simulink model "smib_attack_v2"  (Simulink 8.9)
settings: Solver=ode45  StartTime=0.0  StopTime=10  RelTol=1e-3  EnableMultiTasking=on
values from neighbouring files (symbols this model uses):
  delta0 = 1.1198    [smib_execution.m]
  omega0 = 0    [smib_execution.m]
libraries: simulink x1
settings Model: Creator=Luan Nguyen  LastModifiedBy=LuanNguyen
settings OptimizationCC: ExpressionDepthLimit=2147483647
settings DebuggingCC: MultiTaskDSMMsg=warning  MultiTaskCondExecSysMsg=none  FcnCallInpInsideContextMsg=error
settings GRTTargetCC: CombineOutputUpdateFcns=on  GRTInterface=off
settings ConfigComp: CovSFcnEnable=off

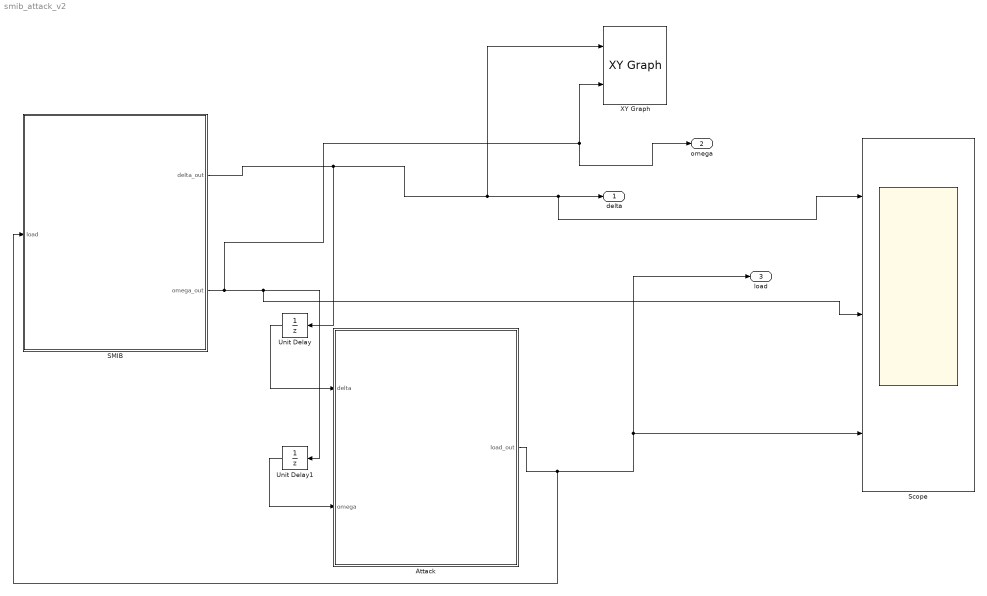
== system smib_attack_v2 ==
  Attack : Stateflow chart  TreatAsAtomicUnit=on
  SMIB : Stateflow chart  TreatAsAtomicUnit=on
  Scope : Scope  NumInputPorts=3
  Unit Delay : UnitDelay  SampleTime=1/100
  Unit Delay1 : UnitDelay  SampleTime=1/100
  XY Graph : simulink/Sinks/XY Graph  xmin=-1  xmax=5  ymin=-2  ymax=5  st=-1
  delta : Outport
  omega : Outport  Port=2
  load : Outport  Port=3
  wires:
  SMIB/1(delta_out) -> Unit Delay/1, XY Graph/1, Scope/1, delta/1
  SMIB/2(omega_out) -> Scope/2, Unit Delay1/1, XY Graph/2, omega/1
  Attack/1(load_out) -> SMIB/1(load), Scope/3, load/1
  Unit Delay/1 -> Attack/1(delta)
  Unit Delay1/1 -> Attack/2(omega)

== stateflow chart SMIB ==
  settings: updateMethod=CONTINUOUS
  state Plant_1
    du:
    delta_dot = omega;
    omega_dot = 9 -10*sin(delta) - omega;
    delta_out = delta;
    omega_out = omega;
  state Plant_2
    du:
    delta_dot = omega;
    omega_dot = -10*sin(delta) - omega;
    delta_out = delta;
    omega_out = omega;
  (default) -> Plant_1 : { omega = omega0; delta = delta0; }
  Plant_1 -> Plant_2 : [load == 1]
  Plant_2 -> Plant_1 : [load == 0]
  data: delta_out output double; omega_out output double; delta local double; omega local double; delta0 local double; omega0 local double; load input double
  data delta settings: updateMethod=SF_CONTINUOUS_TIME_DATA
  data omega settings: updateMethod=SF_CONTINUOUS_TIME_DATA
  data delta0 settings: updateMethod=SF_CONTINUOUS_TIME_DATA
  data omega0 settings: updateMethod=SF_CONTINUOUS_TIME_DATA
  data load settings: updateMethod=SF_CONTINUOUS_TIME_DATA

== stateflow chart Attack ==
  settings: updateMethod=CONTINUOUS
  state Mode1
    du:
    t_dot = 1;
  state Mode2
    du:
    t_dot = 1;
  Mode1 -> Mode2 [order 2] : [delta + omega >= 0.2]
      | {load_out = 1;}
  Mode1 -> Mode2 [order 1] : [delta + omega >= 0.2&&t >=2.5]
      | {load_out = 0;}
  Mode2 -> Mode1 : [delta + omega < -0.2]
      | {load_out = 0;}
  (default) -> Mode1
  data: t local double; load_out output double; delta input double; omega input double
  data t settings: updateMethod=SF_CONTINUOUS_TIME_DATA
  data delta settings: updateMethod=SF_CONTINUOUS_TIME_DATA
  data omega settings: updateMethod=SF_CONTINUOUS_TIME_DATA
